simulink model "untitled"  (Simulink 7.7)
settings: Solver=ode45  StartTime=0.0  StopTime=10.0  RelTol=1e-3
settings Model: Creator=Felipe  LastModifiedBy=Felipe

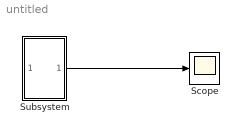
== system untitled ==
  Scope : Scope
  Subsystem : Subsystem
  wires:
  Subsystem/1(Out1) -> Scope/1

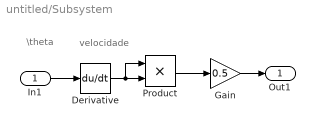
== system untitled/Subsystem ==
  note: \theta
  note: velocidade
  In1 : Inport
  Derivative : Derivative
  Gain : Gain  Gain=0.5
  Product : Product  RndMeth=Zero
  Out1 : Outport
  wires:
  Derivative/1 -> Product/2, Product/1
  Product/1 -> Gain/1
  Gain/1 -> Out1/1
  In1/1 -> Derivative/1
